simulink model "test_direct"  (R2024a)
settings: Solver=VariableStepAuto  StartTime=0.0  StopTime=40  RelTol=1e-3
libraries: neural x733, simulink x4
(part 8 of 35)

== system test_direct/Function Fitting Neural Network/Layer 4/Delays 1 ==
  "p{4}" : Inport  PortDimensions=20
      mask Display: e = 0.06;c1 = [120 230 180]/255;c2 = ([120 230 180]+0)/(256+128);c3 = ([120 230 180]+128)/(256+128);patch([0 1 1 0],[0 0 1 1],c1);patch([0 1 1 1-e 1-e 0+e],[0 0 1 1-e 0+e 0+e],c2);patch([0 0 1 1-e 0+e 0+e],[0 1 1 1-e 1-e 0+e],c3);plot([0 1 1 0 0],[0 0 1 1 0]);
  mux : Mux  Inputs=1
      mask Display: e = 0.06;c1 = [120 150 230]/255;c2 = ([120 150 230]+0)/383;c3 = ([120 150 230]+128)/383;patch([0 1 1 0],[0 0 1 1],c1);patch([0 1 1 1-e 1-e 0+e],[0 0 1 1-e 0+e 0+e],c2);patch([0 0 1 1-e 0+e 0+e],[0 1 1 1-e 1-e 0+e],c3);plot([0 1 1 0 0],[0 0 1 1 0]);disp('Mux')
  "pd{4,3}" : Outport
      mask Display: e = 0.06;c1 = [120 230 180]/255;c2 = ([120 230 180]+0)/(256+128);c3 = ([120 230 180]+128)/(256+128);patch([0 1 1 0],[0 0 1 1],c1);patch([0 1 1 1-e 1-e 0+e],[0 0 1 1-e 0+e 0+e],c2);patch([0 0 1 1-e 0+e 0+e],[0 1 1 1-e 1-e 0+e],c3);plot([0 1 1 0 0],[0 0 1 1 0]);
  wires:
  "p{4}"/1 -> mux/1
  mux/1 -> "pd{4,3}"/1

== system test_direct/Function Fitting Neural Network/Layer 4/LW{4,3} ==
  "ad{4,3}" : Inport  PortDimensions=20
      mask Display: e = 0.06;c1 = [120 230 180]/255;c2 = ([120 230 180]+0)/(256+128);c3 = ([120 230 180]+128)/(256+128);patch([0 1 1 0],[0 0 1 1],c1);patch([0 1 1 1-e 1-e 0+e],[0 0 1 1-e 0+e 0+e],c2);patch([0 0 1 1-e 0+e 0+e],[0 1 1 1-e 1-e 0+e],c3);plot([0 1 1 0 0],[0 0 1 1 0]);
  "IW{4,3}(1,:)'" : Constant  Value=[-0.0182808475685428926948983274769489071331918239593505859375;0.0804580234912133374081122383358888328075408935546875;-0.2073100011052473601314005691165220923721790313720703125;-0.56877624107405078124344299794756807386875152587890625;-0.37106551095573958587436891320976428687572479248046875;0.2453467469113256027579694773521623574197292327880859375;-0.1097157740776300016705135931260883808135986328125;0.293030747380307599048165911881369538605213165283203125;0.4286556952932023545344009107793681323528289794921875;-0.2927619933728118351012881248607300221920013427734375;-0.330831802187190826547436017790460027754306793212890625;-0.01300416253790542993329371057598109473474323749542236328125;-0.220024597925029985479028482586727477610111236572265625;0.28856741284184350693209353266865946352481842041015625;0.1738140495019694087286410422166227363049983978271484375;0.57653717402246307255353485743398778140544891357421875;-0.08144393527626341000580367790462332777678966522216796875;0.62386015914583803354531710283481515944004058837890625;0.23299635893419512466806509110028855502605438232421875;0.462827846568813539018805158775649033486843109130859375]
      mask Display: e = 0.06;c1 = [120 150 230]/255;c2 = ([120 150 230]+0)/383;c3 = ([120 150 230]+128)/383;patch([0 1 1 0],[0 0 1 1],c1);patch([0 1 1 1-e 1-e 0+e],[0 0 1 1-e 0+e 0+e],c2);patch([0 0 1 1-e 0+e 0+e],[0 1 1 1-e 1-e 0+e],c3);plot([0 1 1 0 0],[0 0 1 1 0]);disp('weights');
  "IW{4,3}(10,:)'" : Constant  Value=[-0.5867021051616487792301768422476015985012054443359375;-0.40646884911088843050919194865855388343334197998046875;0.1384930279966194444085658687981776893138885498046875;0.60431005202610743598512499374919570982456207275390625;0.231549088394502333709823460594634525477886199951171875;-0.278578383513912342106522146423230879008769989013671875;-0.2401723445859841599148154500653618015348911285400390625;-0.278682695857914330961335735992179252207279205322265625;0.389949189397055973049788235584856010973453521728515625;-0.378849241372464284882681795352254994213581085205078125;-0.50446895043893802412782179089845158159732818603515625;-0.04123499520558514264134686300167231820523738861083984375;-0.412512646032147267671774670816375873982906341552734375;0.0298074784018579376498880861845464096404612064361572265625;-0.6030020171920196236925448829424567520618438720703125;-0.0918971849790183037409718735943897627294063568115234375;-0.1048877360115925416739202091775950975716114044189453125;0.426138672134914464617594376250053755939006805419921875;-0.028373006982034938705528048785708961077034473419189453125;-0.10103546567123274091404283581141498871147632598876953125]
      mask Display: e = 0.06;c1 = [120 150 230]/255;c2 = ([120 150 230]+0)/383;c3 = ([120 150 230]+128)/383;patch([0 1 1 0],[0 0 1 1],c1);patch([0 1 1 1-e 1-e 0+e],[0 0 1 1-e 0+e 0+e],c2);patch([0 0 1 1-e 0+e 0+e],[0 1 1 1-e 1-e 0+e],c3);plot([0 1 1 0 0],[0 0 1 1 0]);disp('weights');
  "IW{4,3}(2,:)'" : Constant  Value=[0.04766233737430193573292314113132306374609470367431640625;0.472662950403235637697463289441657252609729766845703125;0.393481975518174265094017982846708036959171295166015625;-0.4054200644776970730021048439084552228450775146484375;0.64596436275341506672020841506309807300567626953125;0.34833116550052078963517487864010035991668701171875;0.0158927016381227755037475191102203098125755786895751953125;0.1432191124397620696218069724636734463274478912353515625;-0.1525863659129366445288411568981246091425418853759765625;-0.08213514792309771495038006605682312510907649993896484375;-0.05352653335257491484799885483880643732845783233642578125;-0.2237879229032577743652154822484590113162994384765625;-0.251639048104404128292088671514648012816905975341796875;0.374060271638200159127762844946119002997875213623046875;-0.13843849114586415094407811920973472297191619873046875;-0.00157935386633405584581868463800446988898329436779022216796875;0.08123459901137251859548626953255734406411647796630859375;-0.60194027599860344679427726077847182750701904296875;-0.2419573839009540316968838169486843980848789215087890625;0.4202479369474840797948900217306800186634063720703125]
      mask Display: e = 0.06;c1 = [120 150 230]/255;c2 = ([120 150 230]+0)/383;c3 = ([120 150 230]+128)/383;patch([0 1 1 0],[0 0 1 1],c1);patch([0 1 1 1-e 1-e 0+e],[0 0 1 1-e 0+e 0+e],c2);patch([0 0 1 1-e 0+e 0+e],[0 1 1 1-e 1-e 0+e],c3);plot([0 1 1 0 0],[0 0 1 1 0]);disp('weights');
  "IW{4,3}(3,:)'" : Constant  Value=[0.64653136532270083502993429647176526486873626708984375;-0.17598643231509558670921933298814110457897186279296875;-0.3306166204372065209327047341503202915191650390625;0.5500686330664434908754856223822571337223052978515625;-0.258915156366846421764904562223819084465503692626953125;-0.2135157354375183669237259209694457240402698516845703125;0.0280209258454371910873614837100831209681928157806396484375;0.023128965179387513118047792204379220493137836456298828125;0.300633725443321286885378640363342128694057464599609375;0.34519443371440450274434397215372882783412933349609375;-0.307061664525679400838953370111994445323944091796875;0.0201426192713053155147751027698177495039999485015869140625;0.1928095450190112358779259693619678728282451629638671875;-0.2828180192111175994540417377720586955547332763671875;0.67880942307011460368215693961246870458126068115234375;-0.18199528762274497228901282142032869160175323486328125;0.15160314165136490327512319709057919681072235107421875;0.48788420536031595897696888641803525388240814208984375;0.1995805530883998091251640971677261404693126678466796875;-0.39812724429761658928583756278385408222675323486328125]
      mask Display: e = 0.06;c1 = [120 150 230]/255;c2 = ([120 150 230]+0)/383;c3 = ([120 150 230]+128)/383;patch([0 1 1 0],[0 0 1 1],c1);patch([0 1 1 1-e 1-e 0+e],[0 0 1 1-e 0+e 0+e],c2);patch([0 0 1 1-e 0+e 0+e],[0 1 1 1-e 1-e 0+e],c3);plot([0 1 1 0 0],[0 0 1 1 0]);disp('weights');
  "IW{4,3}(4,:)'" : Constant  Value=[0.46897639649297795383375841993256472051143646240234375;0.1353316784521863269663555229271878488361835479736328125;-0.4090318643737698156570559149258770048618316650390625;-0.10034667176648993935916820419151918031275272369384765625;0.15356197843960306403943150144186802208423614501953125;-0.74982192036332262485842647947720251977443695068359375;0.736163475218127860699723896686919033527374267578125;-0.388099606476475178507001828620559535920619964599609375;0.1284378189965413030737551025595166720449924468994140625;-0.35342224141770184342448146708193235099315643310546875;0.33768468281888275317470515801687724888324737548828125;-0.33768459631601943637946305898367427289485931396484375;0.339246448835974323543496211641468107700347900390625;-0.182148817954333519519849460266414098441600799560546875;-0.45675022943742826786461819210671819746494293212890625;-0.1308331396638943433519131076536723412573337554931640625;0.007235920518857773438281544287065116805024445056915283203125;-0.2181989741993194120706078820148832164704799652099609375;0.697710740419517083665823520277626812458038330078125;0.03270757109621826030920743733076960779726505279541015625]
      mask Display: e = 0.06;c1 = [120 150 230]/255;c2 = ([120 150 230]+0)/383;c3 = ([120 150 230]+128)/383;patch([0 1 1 0],[0 0 1 1],c1);patch([0 1 1 1-e 1-e 0+e],[0 0 1 1-e 0+e 0+e],c2);patch([0 0 1 1-e 0+e 0+e],[0 1 1 1-e 1-e 0+e],c3);plot([0 1 1 0 0],[0 0 1 1 0]);disp('weights');
  "IW{4,3}(5,:)'" : Constant  Value=[0.254012415241254452258345963855390436947345733642578125;-0.278201611801674075774570837893406860530376434326171875;-0.130987915740999272262712338488199748098850250244140625;0.65659498971948615508864577350323088467121124267578125;-0.37010577209780526342086659496999345719814300537109375;-0.364239904557088711722911966717219911515712738037109375;-0.346218175332081823381003005124512128531932830810546875;-0.131514115645591733727570726841804571449756622314453125;-0.16293218459890457250338613448548130691051483154296875;-0.07690950801719813323398255988649907521903514862060546875;-0.04995568746558680384151074349574628286063671112060546875;-0.297894174787131815751450858442694880068302154541015625;-0.208190351516119920294300982277491129934787750244140625;-0.13629072817438714348980965951341204345226287841796875;-0.384110184134717147497184441817807964980602264404296875;-0.43900730118536801516171408366062678396701812744140625;0.0692901289663383213035530161505448631942272186279296875;0.27697027123827278050072209225618280470371246337890625;0.0208057391676239288036409647020263946615159511566162109375;0.6856311827603163155941956574679352343082427978515625]
      mask Display: e = 0.06;c1 = [120 150 230]/255;c2 = ([120 150 230]+0)/383;c3 = ([120 150 230]+128)/383;patch([0 1 1 0],[0 0 1 1],c1);patch([0 1 1 1-e 1-e 0+e],[0 0 1 1-e 0+e 0+e],c2);patch([0 0 1 1-e 0+e 0+e],[0 1 1 1-e 1-e 0+e],c3);plot([0 1 1 0 0],[0 0 1 1 0]);disp('weights');
  "IW{4,3}(6,:)'" : Constant  Value=[0.06383515321962386634968567022951901890337467193603515625;-0.348969499010585881837442912001279182732105255126953125;-0.67269644646642923202506381130660884082317352294921875;0.44685601061213520157622269834973849356174468994140625;-0.358281232233862712011074336260207928717136383056640625;0.07916658582745154937310161358254845254123210906982421875;0.30505773608176711686468252082704566419124603271484375;0.617951579143801499327537385397590696811676025390625;-0.25294218554518221875326844383380375802516937255859375;-0.3977997598759459574324637287645600736141204833984375;0.058739564042513479902307693691909662447869777679443359375;0.1494537664697459522500366801978088915348052978515625;0.60851330942889114705707243047072552144527435302734375;-0.055559362022579848738867980273425928317010402679443359375;-0.62443423379172180442964190660859458148479461669921875;-0.2268644620133335454426060096011497080326080322265625;-0.57816378248105604331641416138154454529285430908203125;0.39207408987547409662255404327879659831523895263671875;-0.074342103653326108148036155398585833609104156494140625;0.285697237530900871593786405355785973370075225830078125]
      mask Display: e = 0.06;c1 = [120 150 230]/255;c2 = ([120 150 230]+0)/383;c3 = ([120 150 230]+128)/383;patch([0 1 1 0],[0 0 1 1],c1);patch([0 1 1 1-e 1-e 0+e],[0 0 1 1-e 0+e 0+e],c2);patch([0 0 1 1-e 0+e 0+e],[0 1 1 1-e 1-e 0+e],c3);plot([0 1 1 0 0],[0 0 1 1 0]);disp('weights');
  "IW{4,3}(7,:)'" : Constant  Value=[0.1735578250848583692356186247707228176295757293701171875;-0.1443796965013408317712872985794092528522014617919921875;-0.00192713703805364963174417969327123500988818705081939697265625;-0.050944766962450170610932076442622928880155086517333984375;-0.56313960947635821607804018640308640897274017333984375;0.406795735506861155794666728979791514575481414794921875;-0.43477191912486556901740186731331050395965576171875;-0.0183635163924778209432187026095562032423913478851318359375;-0.16499808196158738393677367639611475169658660888671875;0.1554097258561016603461979457279085181653499603271484375;-0.45712271023931894120551078231073915958404541015625;-0.31639810290967407269135946989990770816802978515625;0.283675985048455980841453083485248498618602752685546875;-0.434852696669257132722208325503743253648281097412109375;0.184268928265691245282908994340687058866024017333984375;0.487799544058790834899497212973074056208133697509765625;-0.1646897501250245976489594568192842416465282440185546875;0.55969685707381255923564822296611964702606201171875;-0.40425367209081686237226449520676396787166595458984375;0.259423740372571154377823177128448151051998138427734375]
      mask Display: e = 0.06;c1 = [120 150 230]/255;c2 = ([120 150 230]+0)/383;c3 = ([120 150 230]+128)/383;patch([0 1 1 0],[0 0 1 1],c1);patch([0 1 1 1-e 1-e 0+e],[0 0 1 1-e 0+e 0+e],c2);patch([0 0 1 1-e 0+e 0+e],[0 1 1 1-e 1-e 0+e],c3);plot([0 1 1 0 0],[0 0 1 1 0]);disp('weights');
  "IW{4,3}(8,:)'" : Constant  Value=[-0.044604630833756091223829542968815076164901256561279296875;0.1653273492054885551727494430451770313084125518798828125;0.35228947713259184393308487415197305381298065185546875;0.388185803066177392839364301835303194820880889892578125;0.59881679713870406001063884104951284825801849365234375;-0.07736001152979880834958947843915666453540325164794921875;-0.5271011175306501428394767572171986103057861328125;-0.09774032952107626626148118020864785648882389068603515625;0.18675638954029449845251065198681317269802093505859375;-0.478571423377917526398306335977395065128803253173828125;0.34027059434836159912407538286061026155948638916015625;0.057705036219698628563445907957429881207644939422607421875;-0.214782881199087782864154405615408904850482940673828125;-0.26706306507587018739258155619609169661998748779296875;-0.54002602442711433727851044750423170626163482666015625;0.58528571806826767964793134524370543658733367919921875;0.030194751746646243673044551769635290838778018951416015625;-0.4346282259921803170499288171413354575634002685546875;0.40357189348227062719587365791085176169872283935546875;0.193904249336287748395335484019597060978412628173828125]
      mask Display: e = 0.06;c1 = [120 150 230]/255;c2 = ([120 150 230]+0)/383;c3 = ([120 150 230]+128)/383;patch([0 1 1 0],[0 0 1 1],c1);patch([0 1 1 1-e 1-e 0+e],[0 0 1 1-e 0+e 0+e],c2);patch([0 0 1 1-e 0+e 0+e],[0 1 1 1-e 1-e 0+e],c3);plot([0 1 1 0 0],[0 0 1 1 0]);disp('weights');
  "IW{4,3}(9,:)'" : Constant  Value=[-0.262696724536377546055376797085045836865901947021484375;-0.495272708083491608466175648572971113026142120361328125;-0.3543852059837149237608855401049368083477020263671875;-0.221393523730061769771992885580402798950672149658203125;-0.038436478394411034698041618185015977360308170318603515625;-0.318611608590077199920642669894732534885406494140625;-0.07339652443837078876764934420862118713557720184326171875;1.061095964250348355761843777145259082317352294921875;-0.4127361165109009188967092995881102979183197021484375;-0.025399426654827285398940972527270787395536899566650390625;-0.5236953508005728341601070496835745871067047119140625;-0.335822568857687187016125562877277843654155731201171875;0.350185935701288586496815469217835925519466400146484375;-0.195141267318745648129407754822750575840473175048828125;0.9131446131154741241431338494294323027133941650390625;-0.4326775227891754838083215872757136821746826171875;-0.63697775880777218748818313542869873344898223876953125;0.55100216042612715217074992324342019855976104736328125;-0.09919080628567943092033232233006856404244899749755859375;0.134968530413840992476792735033086501061916351318359375]
      mask Display: e = 0.06;c1 = [120 150 230]/255;c2 = ([120 150 230]+0)/383;c3 = ([120 150 230]+128)/383;patch([0 1 1 0],[0 0 1 1],c1);patch([0 1 1 1-e 1-e 0+e],[0 0 1 1-e 0+e 0+e],c2);patch([0 0 1 1-e 0+e 0+e],[0 1 1 1-e 1-e 0+e],c3);plot([0 1 1 0 0],[0 0 1 1 0]);disp('weights');
  Mux : Mux  Inputs=10
      mask Display: e = 0.06;c1 = [120 150 230]/255;c2 = ([120 150 230]+0)/383;c3 = ([120 150 230]+128)/383;patch([0 1 1 0],[0 0 1 1],c1);patch([0 1 1 1-e 1-e 0+e],[0 0 1 1-e 0+e 0+e],c2);patch([0 0 1 1-e 0+e 0+e],[0 1 1 1-e 1-e 0+e],c3);plot([0 1 1 0 0],[0 0 1 1 0]);disp('Mux');
  dotprod{1..10} (10 alike) : neural/Weight Functions/dotprod
  "lz{4,3}" : Outport
      mask Display: e = 0.06;c1 = [120 230 180]/255;c2 = ([120 230 180]+0)/(256+128);c3 = ([120 230 180]+128)/(256+128);patch([0 1 1 0],[0 0 1 1],c1);patch([0 1 1 1-e 1-e 0+e],[0 0 1 1-e 0+e 0+e],c2);patch([0 0 1 1-e 0+e 0+e],[0 1 1 1-e 1-e 0+e],c3);plot([0 1 1 0 0],[0 0 1 1 0]);
  wires:
  "IW{4,3}(1,:)'"/1 -> dotprod1/1
  "ad{4,3}"/1 -> dotprod1/2, dotprod2/2, dotprod3/2, dotprod4/2, dotprod5/2, dotprod6/2, dotprod7/2, dotprod8/2, dotprod9/2, dotprod10/2
  dotprod1/1 -> Mux/1
  "IW{4,3}(2,:)'"/1 -> dotprod2/1
  dotprod2/1 -> Mux/2
  "IW{4,3}(3,:)'"/1 -> dotprod3/1
  dotprod3/1 -> Mux/3
  "IW{4,3}(4,:)'"/1 -> dotprod4/1
  dotprod4/1 -> Mux/4
  "IW{4,3}(5,:)'"/1 -> dotprod5/1
  dotprod5/1 -> Mux/5
  "IW{4,3}(6,:)'"/1 -> dotprod6/1
  dotprod6/1 -> Mux/6
  "IW{4,3}(7,:)'"/1 -> dotprod7/1
  dotprod7/1 -> Mux/7
  "IW{4,3}(8,:)'"/1 -> dotprod8/1
  dotprod8/1 -> Mux/8
  "IW{4,3}(9,:)'"/1 -> dotprod9/1
  dotprod9/1 -> Mux/9
  "IW{4,3}(10,:)'"/1 -> dotprod10/1
  dotprod10/1 -> Mux/10
  Mux/1 -> "lz{4,3}"/1

== system test_direct/Function Fitting Neural Network/Layer 5/Delays 1 ==
  "p{5}" : Inport  PortDimensions=10
      mask Display: e = 0.06;c1 = [120 230 180]/255;c2 = ([120 230 180]+0)/(256+128);c3 = ([120 230 180]+128)/(256+128);patch([0 1 1 0],[0 0 1 1],c1);patch([0 1 1 1-e 1-e 0+e],[0 0 1 1-e 0+e 0+e],c2);patch([0 0 1 1-e 0+e 0+e],[0 1 1 1-e 1-e 0+e],c3);plot([0 1 1 0 0],[0 0 1 1 0]);
  mux : Mux  Inputs=1
      mask Display: e = 0.06;c1 = [120 150 230]/255;c2 = ([120 150 230]+0)/383;c3 = ([120 150 230]+128)/383;patch([0 1 1 0],[0 0 1 1],c1);patch([0 1 1 1-e 1-e 0+e],[0 0 1 1-e 0+e 0+e],c2);patch([0 0 1 1-e 0+e 0+e],[0 1 1 1-e 1-e 0+e],c3);plot([0 1 1 0 0],[0 0 1 1 0]);disp('Mux')
  "pd{5,4}" : Outport
      mask Display: e = 0.06;c1 = [120 230 180]/255;c2 = ([120 230 180]+0)/(256+128);c3 = ([120 230 180]+128)/(256+128);patch([0 1 1 0],[0 0 1 1],c1);patch([0 1 1 1-e 1-e 0+e],[0 0 1 1-e 0+e 0+e],c2);patch([0 0 1 1-e 0+e 0+e],[0 1 1 1-e 1-e 0+e],c3);plot([0 1 1 0 0],[0 0 1 1 0]);
  wires:
  "p{5}"/1 -> mux/1
  mux/1 -> "pd{5,4}"/1

== system test_direct/Function Fitting Neural Network/Layer 5/LW{5,4} ==
  "ad{5,4}" : Inport  PortDimensions=10
      mask Display: e = 0.06;c1 = [120 230 180]/255;c2 = ([120 230 180]+0)/(256+128);c3 = ([120 230 180]+128)/(256+128);patch([0 1 1 0],[0 0 1 1],c1);patch([0 1 1 1-e 1-e 0+e],[0 0 1 1-e 0+e 0+e],c2);patch([0 0 1 1-e 0+e 0+e],[0 1 1 1-e 1-e 0+e],c3);plot([0 1 1 0 0],[0 0 1 1 0]);
  "IW{5,4}(1,:)'" : Constant  Value=[-0.609586613853234648985335297766141593456268310546875;-0.991992343621268535258650445030070841312408447265625;0.55645920623334166332796257847803644835948944091796875;-0.2756548382209949021870443175430409610271453857421875;0.79182679604217509616859160814783535897731781005859375;0.5409353217326822171884259660146199166774749755859375;0.8560146531317720519638214682345278561115264892578125;0.369094621261524424848943226606934331357479095458984375;1.144450010398711636838697813800536096096038818359375;0.82688754328264491011424297539633698761463165283203125]
      mask Display: e = 0.06;c1 = [120 150 230]/255;c2 = ([120 150 230]+0)/383;c3 = ([120 150 230]+128)/383;patch([0 1 1 0],[0 0 1 1],c1);patch([0 1 1 1-e 1-e 0+e],[0 0 1 1-e 0+e 0+e],c2);patch([0 0 1 1-e 0+e 0+e],[0 1 1 1-e 1-e 0+e],c3);plot([0 1 1 0 0],[0 0 1 1 0]);disp('weights');
  "IW{5,4}(2,:)'" : Constant  Value=[-0.2491134788551136736156621509508113376796245574951171875;-0.348638402621329834829566607368178665637969970703125;-0.58928454736647262190984974949969910085201263427734375;1.1057017527083596863946013399981893599033355712890625;0.69839147102565746205726782136480323970317840576171875;-0.78717405206411239504404875333420932292938232421875;0.1763952297557981607756261155373067595064640045166015625;-0.0641150518456101436992611297682742588222026824951171875;-0.9062580556750947646804661417263559997081756591796875;-1.0565207862803387417471867593121714890003204345703125]
      mask Display: e = 0.06;c1 = [120 150 230]/255;c2 = ([120 150 230]+0)/383;c3 = ([120 150 230]+128)/383;patch([0 1 1 0],[0 0 1 1],c1);patch([0 1 1 1-e 1-e 0+e],[0 0 1 1-e 0+e 0+e],c2);patch([0 0 1 1-e 0+e 0+e],[0 1 1 1-e 1-e 0+e],c3);plot([0 1 1 0 0],[0 0 1 1 0]);disp('weights');
  Mux : Mux  Inputs=2
      mask Display: e = 0.06;c1 = [120 150 230]/255;c2 = ([120 150 230]+0)/383;c3 = ([120 150 230]+128)/383;patch([0 1 1 0],[0 0 1 1],c1);patch([0 1 1 1-e 1-e 0+e],[0 0 1 1-e 0+e 0+e],c2);patch([0 0 1 1-e 0+e 0+e],[0 1 1 1-e 1-e 0+e],c3);plot([0 1 1 0 0],[0 0 1 1 0]);disp('Mux');
  dotprod1 : neural/Weight Functions/dotprod
  dotprod2 : neural/Weight Functions/dotprod
  "lz{5,4}" : Outport
      mask Display: e = 0.06;c1 = [120 230 180]/255;c2 = ([120 230 180]+0)/(256+128);c3 = ([120 230 180]+128)/(256+128);patch([0 1 1 0],[0 0 1 1],c1);patch([0 1 1 1-e 1-e 0+e],[0 0 1 1-e 0+e 0+e],c2);patch([0 0 1 1-e 0+e 0+e],[0 1 1 1-e 1-e 0+e],c3);plot([0 1 1 0 0],[0 0 1 1 0]);
  wires:
  "IW{5,4}(1,:)'"/1 -> dotprod1/1
  "ad{5,4}"/1 -> dotprod1/2, dotprod2/2
  dotprod1/1 -> Mux/1
  "IW{5,4}(2,:)'"/1 -> dotprod2/1
  dotprod2/1 -> Mux/2
  Mux/1 -> "lz{5,4}"/1

== system test_direct/Function Fitting Neural Network1/Layer 1/Delays 1 ==
  "p{1}" : Inport  PortDimensions=8
      mask Display: e = 0.06;c1 = [120 230 180]/255;c2 = ([120 230 180]+0)/(256+128);c3 = ([120 230 180]+128)/(256+128);patch([0 1 1 0],[0 0 1 1],c1);patch([0 1 1 1-e 1-e 0+e],[0 0 1 1-e 0+e 0+e],c2);patch([0 0 1 1-e 0+e 0+e],[0 1 1 1-e 1-e 0+e],c3);plot([0 1 1 0 0],[0 0 1 1 0]);
  mux : Mux  Inputs=1
      mask Display: e = 0.06;c1 = [120 150 230]/255;c2 = ([120 150 230]+0)/383;c3 = ([120 150 230]+128)/383;patch([0 1 1 0],[0 0 1 1],c1);patch([0 1 1 1-e 1-e 0+e],[0 0 1 1-e 0+e 0+e],c2);patch([0 0 1 1-e 0+e 0+e],[0 1 1 1-e 1-e 0+e],c3);plot([0 1 1 0 0],[0 0 1 1 0]);disp('Mux')
  "pd{1,1}" : Outport
      mask Display: e = 0.06;c1 = [120 230 180]/255;c2 = ([120 230 180]+0)/(256+128);c3 = ([120 230 180]+128)/(256+128);patch([0 1 1 0],[0 0 1 1],c1);patch([0 1 1 1-e 1-e 0+e],[0 0 1 1-e 0+e 0+e],c2);patch([0 0 1 1-e 0+e 0+e],[0 1 1 1-e 1-e 0+e],c3);plot([0 1 1 0 0],[0 0 1 1 0]);
  wires:
  "p{1}"/1 -> mux/1
  mux/1 -> "pd{1,1}"/1

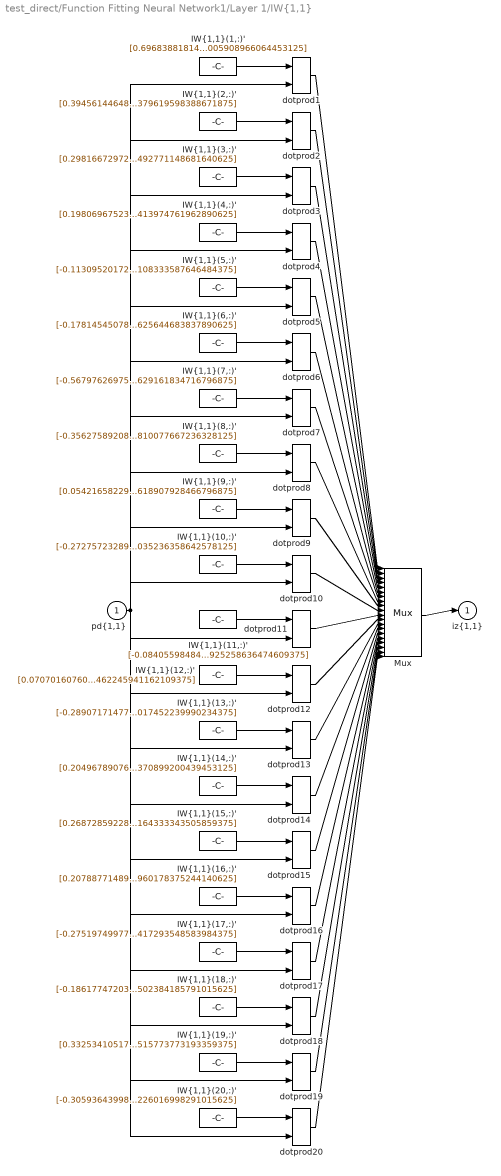
== system test_direct/Function Fitting Neural Network1/Layer 1/IW{1,1} ==
  "pd{1,1}" : Inport  PortDimensions=8
      mask Display: e = 0.06;c1 = [120 230 180]/255;c2 = ([120 230 180]+0)/(256+128);c3 = ([120 230 180]+128)/(256+128);patch([0 1 1 0],[0 0 1 1],c1);patch([0 1 1 1-e 1-e 0+e],[0 0 1 1-e 0+e 0+e],c2);patch([0 0 1 1-e 0+e 0+e],[0 1 1 1-e 1-e 0+e],c3);plot([0 1 1 0 0],[0 0 1 1 0]);
  "IW{1,1}(1,:)'" : Constant  Value=[0.69683881814263559650868273820378817617893218994140625;0.7640431505441267479028510933858342468738555908203125;0.67792814742460449917160758559475652873516082763671875;-0.564455292301047517611323200981132686138153076171875;0.0206524861164411911718108427749029942788183689117431640625;0.63667859510223190344646582161658443510532379150390625;1.00234633248641813452195492573082447052001953125;0.05889755968272869512958322957274504005908966064453125]
      mask Display: e = 0.06;c1 = [120 150 230]/255;c2 = ([120 150 230]+0)/383;c3 = ([120 150 230]+128)/383;patch([0 1 1 0],[0 0 1 1],c1);patch([0 1 1 1-e 1-e 0+e],[0 0 1 1-e 0+e 0+e],c2);patch([0 0 1 1-e 0+e 0+e],[0 1 1 1-e 1-e 0+e],c3);plot([0 1 1 0 0],[0 0 1 1 0]);disp('Weights');
  "IW{1,1}(10,:)'" : Constant  Value=[-0.272757232895687706797360760901938192546367645263671875;-0.26724039829289625291863785605528391897678375244140625;0.07275557598798353120539417204781784676015377044677734375;-0.2024513959855038514046299269466544501483440399169921875;0.3419638465162890827997443921049125492572784423828125;1.33460318464404448235427480540238320827484130859375;-0.0387887916615675398812612684196210466325283050537109375;0.213400994483100625576099673708085902035236358642578125]
      mask Display: e = 0.06;c1 = [120 150 230]/255;c2 = ([120 150 230]+0)/383;c3 = ([120 150 230]+128)/383;patch([0 1 1 0],[0 0 1 1],c1);patch([0 1 1 1-e 1-e 0+e],[0 0 1 1-e 0+e 0+e],c2);patch([0 0 1 1-e 0+e 0+e],[0 1 1 1-e 1-e 0+e],c3);plot([0 1 1 0 0],[0 0 1 1 0]);disp('Weights');
  "IW{1,1}(11,:)'" : Constant  Value=[-0.08405598484492704525194994857884012162685394287109375;0.22475151025755268907602157923975028097629547119140625;0.515237557803050805205202777869999408721923828125;0.362218047367421858151459446162334643304347991943359375;0.6853072384581058162922317933407612144947052001953125;0.49951312939876679752870813899789936840534210205078125;0.30454149529149532327210181392729282379150390625;-1.2259255997811100424854657831019721925258636474609375]
      mask Display: e = 0.06;c1 = [120 150 230]/255;c2 = ([120 150 230]+0)/383;c3 = ([120 150 230]+128)/383;patch([0 1 1 0],[0 0 1 1],c1);patch([0 1 1 1-e 1-e 0+e],[0 0 1 1-e 0+e 0+e],c2);patch([0 0 1 1-e 0+e 0+e],[0 1 1 1-e 1-e 0+e],c3);plot([0 1 1 0 0],[0 0 1 1 0]);disp('Weights');
  "IW{1,1}(12,:)'" : Constant  Value=[0.070701607607360938967389074605307541787624359130859375;0.360937305657575258077685020907665602862834930419921875;-0.54966145677578925887729610622045584022998809814453125;0.57478890048600173034998306320630945265293121337890625;0.5999359439613123345935719044064171612262725830078125;-0.1187698884370364804663466884449007920920848846435546875;-0.98272714657886572897638188806013204157352447509765625;0.3155743205749350632771665914333425462245941162109375]
      mask Display: e = 0.06;c1 = [120 150 230]/255;c2 = ([120 150 230]+0)/383;c3 = ([120 150 230]+128)/383;patch([0 1 1 0],[0 0 1 1],c1);patch([0 1 1 1-e 1-e 0+e],[0 0 1 1-e 0+e 0+e],c2);patch([0 0 1 1-e 0+e 0+e],[0 1 1 1-e 1-e 0+e],c3);plot([0 1 1 0 0],[0 0 1 1 0]);disp('Weights');
  "IW{1,1}(13,:)'" : Constant  Value=[-0.2890717147788859353596535584074445068836212158203125;-0.242197251466092222660364541297894902527332305908203125;0.1863621649756492526517348551351460628211498260498046875;0.5305730473676708580654803881770931184291839599609375;-0.410514280193981451194673581994720734655857086181640625;-0.32544911037928070385305545642040669918060302734375;-0.1853150999010389210486238198427599854767322540283203125;1.117782813867628899373585227294825017452239990234375]
      mask Display: e = 0.06;c1 = [120 150 230]/255;c2 = ([120 150 230]+0)/383;c3 = ([120 150 230]+128)/383;patch([0 1 1 0],[0 0 1 1],c1);patch([0 1 1 1-e 1-e 0+e],[0 0 1 1-e 0+e 0+e],c2);patch([0 0 1 1-e 0+e 0+e],[0 1 1 1-e 1-e 0+e],c3);plot([0 1 1 0 0],[0 0 1 1 0]);disp('Weights');
  "IW{1,1}(14,:)'" : Constant  Value=[0.20496789076231902715363730749231763184070587158203125;0.26429751124447797838712403972749598324298858642578125;0.36484988902725346004984885439625941216945648193359375;-0.5745167996217379613455022990819998085498809814453125;-0.497719456328582554593964459854760207235813140869140625;1.2500259012874488373512349426164291799068450927734375;0.159100403766398112992419555666856467723846435546875;-1.011690432173470544086057998356409370899200439453125]
      mask Display: e = 0.06;c1 = [120 150 230]/255;c2 = ([120 150 230]+0)/383;c3 = ([120 150 230]+128)/383;patch([0 1 1 0],[0 0 1 1],c1);patch([0 1 1 1-e 1-e 0+e],[0 0 1 1-e 0+e 0+e],c2);patch([0 0 1 1-e 0+e 0+e],[0 1 1 1-e 1-e 0+e],c3);plot([0 1 1 0 0],[0 0 1 1 0]);disp('Weights');
  "IW{1,1}(15,:)'" : Constant  Value=[0.268728592282806710844766939771943725645542144775390625;0.3038613381826598125456939669675193727016448974609375;0.289458329765824140533680974840535782277584075927734375;-0.5409659514970897031815866284887306392192840576171875;-0.341031491431749878007195775353466160595417022705078125;0.289089703738018399814535541736404411494731903076171875;-1.0600111717134639288673270129947923123836517333984375;-0.283062967641139306973485645357868634164333343505859375]
      mask Display: e = 0.06;c1 = [120 150 230]/255;c2 = ([120 150 230]+0)/383;c3 = ([120 150 230]+128)/383;patch([0 1 1 0],[0 0 1 1],c1);patch([0 1 1 1-e 1-e 0+e],[0 0 1 1-e 0+e 0+e],c2);patch([0 0 1 1-e 0+e 0+e],[0 1 1 1-e 1-e 0+e],c3);plot([0 1 1 0 0],[0 0 1 1 0]);disp('Weights');
  "IW{1,1}(16,:)'" : Constant  Value=[0.2078877148940026231560551650545676238834857940673828125;0.0840721456582262105516889505452127195894718170166015625;0.4795104000373415775726471110829152166843414306640625;-0.767481223732529027614646111032925546169281005859375;0.45378680057911624512456683078198693692684173583984375;-1.107609818954824465464525928837247192859649658203125;0.0561311271008308187990820670165703631937503814697265625;1.3254891299923559078166590552427805960178375244140625]
      mask Display: e = 0.06;c1 = [120 150 230]/255;c2 = ([120 150 230]+0)/383;c3 = ([120 150 230]+128)/383;patch([0 1 1 0],[0 0 1 1],c1);patch([0 1 1 1-e 1-e 0+e],[0 0 1 1-e 0+e 0+e],c2);patch([0 0 1 1-e 0+e 0+e],[0 1 1 1-e 1-e 0+e],c3);plot([0 1 1 0 0],[0 0 1 1 0]);disp('Weights');
  "IW{1,1}(17,:)'" : Constant  Value=[-0.275197499773989162630272176102153025567531585693359375;-0.44914330240078592648700350764556787908077239990234375;-0.10215451095910664525145961079033440910279750823974609375;-0.336551936442363419654810741121764294803142547607421875;0.1538071143495922943333908960994449444115161895751953125;-0.86003499709754260837968331543379463255405426025390625;-1.1816622408107642083763266782625578343868255615234375;0.6442531105253210821359743931679986417293548583984375]
      mask Display: e = 0.06;c1 = [120 150 230]/255;c2 = ([120 150 230]+0)/383;c3 = ([120 150 230]+128)/383;patch([0 1 1 0],[0 0 1 1],c1);patch([0 1 1 1-e 1-e 0+e],[0 0 1 1-e 0+e 0+e],c2);patch([0 0 1 1-e 0+e 0+e],[0 1 1 1-e 1-e 0+e],c3);plot([0 1 1 0 0],[0 0 1 1 0]);disp('Weights');
  "IW{1,1}(18,:)'" : Constant  Value=[-0.18617747203861301219518509242334403097629547119140625;0.6961684748736256533874211527290754020214080810546875;-0.794298894762984541983996678027324378490447998046875;0.9533966695713740335804686765186488628387451171875;-0.429132320048394466649455125661916099488735198974609375;-0.60641702663512209170448841177858412265777587890625;-0.5869788837731719777224270728765986859798431396484375;-0.67739230044078679870978021426708437502384185791015625]
      mask Display: e = 0.06;c1 = [120 150 230]/255;c2 = ([120 150 230]+0)/383;c3 = ([120 150 230]+128)/383;patch([0 1 1 0],[0 0 1 1],c1);patch([0 1 1 1-e 1-e 0+e],[0 0 1 1-e 0+e 0+e],c2);patch([0 0 1 1-e 0+e 0+e],[0 1 1 1-e 1-e 0+e],c3);plot([0 1 1 0 0],[0 0 1 1 0]);disp('Weights');
  "IW{1,1}(19,:)'" : Constant  Value=[0.332534105179708106003744205736438743770122528076171875;0.1373651819662270179289720317683531902730464935302734375;-0.095512741275323442824429776010219939053058624267578125;-0.92288801670492404127799090929329395294189453125;0.6482460639796414625379838980734348297119140625;0.359576586366763761848375224872143007814884185791015625;0.06857172282922495420987019087988301180303096771240234375;1.3221821932444155489605464026681147515773773193359375]
      mask Display: e = 0.06;c1 = [120 150 230]/255;c2 = ([120 150 230]+0)/383;c3 = ([120 150 230]+128)/383;patch([0 1 1 0],[0 0 1 1],c1);patch([0 1 1 1-e 1-e 0+e],[0 0 1 1-e 0+e 0+e],c2);patch([0 0 1 1-e 0+e 0+e],[0 1 1 1-e 1-e 0+e],c3);plot([0 1 1 0 0],[0 0 1 1 0]);disp('Weights');
  "IW{1,1}(2,:)'" : Constant  Value=[0.394561446481398292451814313608338125050067901611328125;0.496126296863468263520502432584180496633052825927734375;0.456100600010595214062192326309741474688053131103515625;-0.628533744301563501721830107271671295166015625;-0.7743125299354953749997321210685186088085174560546875;1.2798934719664074588507673979620449244976043701171875;0.78492340665270976529654944897629320621490478515625;-0.433530743610808400045897315067122690379619598388671875]
      mask Display: e = 0.06;c1 = [120 150 230]/255;c2 = ([120 150 230]+0)/383;c3 = ([120 150 230]+128)/383;patch([0 1 1 0],[0 0 1 1],c1);patch([0 1 1 1-e 1-e 0+e],[0 0 1 1-e 0+e 0+e],c2);patch([0 0 1 1-e 0+e 0+e],[0 1 1 1-e 1-e 0+e],c3);plot([0 1 1 0 0],[0 0 1 1 0]);disp('Weights');
  "IW{1,1}(20,:)'" : Constant  Value=[-0.30593643998864517019597997204982675611972808837890625;-0.9213158914543253530382571625523269176483154296875;0.7853169865737832378016491929884068667888641357421875;-0.81818362218703821753251759218983352184295654296875;-0.56443628264250544912528084751102142035961151123046875;-0.56868329177563092802216715426766313612461090087890625;-0.32446229273851467933553749389830045402050018310546875;-0.94825291764287611417927337242872454226016998291015625]
      mask Display: e = 0.06;c1 = [120 150 230]/255;c2 = ([120 150 230]+0)/383;c3 = ([120 150 230]+128)/383;patch([0 1 1 0],[0 0 1 1],c1);patch([0 1 1 1-e 1-e 0+e],[0 0 1 1-e 0+e 0+e],c2);patch([0 0 1 1-e 0+e 0+e],[0 1 1 1-e 1-e 0+e],c3);plot([0 1 1 0 0],[0 0 1 1 0]);disp('Weights');
  "IW{1,1}(3,:)'" : Constant  Value=[0.298166729727484425271910595256485976278781890869140625;-0.4183300027243743723914803922525607049465179443359375;-0.80799038393734090579556550437700934708118438720703125;-0.505366820627469959248401210061274468898773193359375;-0.253730462639679188452390690144966356456279754638671875;0.83661243378666227954454370774328708648681640625;-0.78793602729768352777028894706745631992816925048828125;-0.8556624788960223160216855831095017492771148681640625]
      mask Display: e = 0.06;c1 = [120 150 230]/255;c2 = ([120 150 230]+0)/383;c3 = ([120 150 230]+128)/383;patch([0 1 1 0],[0 0 1 1],c1);patch([0 1 1 1-e 1-e 0+e],[0 0 1 1-e 0+e 0+e],c2);patch([0 0 1 1-e 0+e 0+e],[0 1 1 1-e 1-e 0+e],c3);plot([0 1 1 0 0],[0 0 1 1 0]);disp('Weights');
  "IW{1,1}(4,:)'" : Constant  Value=[0.1980696752360057433239859392415382899343967437744140625;0.2404467731306450251071993307050433941185474395751953125;0.1788655051560224806816989939761697314679622650146484375;-0.3289918451008759792131286303629167377948760986328125;0.1697279131019995279672230026335455477237701416015625;-0.437020546507040308359393065984477289021015167236328125;1.00415962486495136118946902570314705371856689453125;1.0487130245760918345609979951404966413974761962890625]
      mask Display: e = 0.06;c1 = [120 150 230]/255;c2 = ([120 150 230]+0)/383;c3 = ([120 150 230]+128)/383;patch([0 1 1 0],[0 0 1 1],c1);patch([0 1 1 1-e 1-e 0+e],[0 0 1 1-e 0+e 0+e],c2);patch([0 0 1 1-e 0+e 0+e],[0 1 1 1-e 1-e 0+e],c3);plot([0 1 1 0 0],[0 0 1 1 0]);disp('Weights');
  "IW{1,1}(5,:)'" : Constant  Value=[-0.1130952017268885001488598618379910476505756378173828125;0.1344070985514231042490251866183825768530368804931640625;-0.76878839995911640858849978030775673687458038330078125;0.297090955023965985759559771395288407802581787109375;0.52419815521998902596578773227520287036895751953125;-0.405912798675867769748748514757608063519001007080078125;0.9627247316031388724155704039731062948703765869140625;0.1682518404063882699883691884679137729108333587646484375]
      mask Display: e = 0.06;c1 = [120 150 230]/255;c2 = ([120 150 230]+0)/383;c3 = ([120 150 230]+128)/383;patch([0 1 1 0],[0 0 1 1],c1);patch([0 1 1 1-e 1-e 0+e],[0 0 1 1-e 0+e 0+e],c2);patch([0 0 1 1-e 0+e 0+e],[0 1 1 1-e 1-e 0+e],c3);plot([0 1 1 0 0],[0 0 1 1 0]);disp('Weights');
  "IW{1,1}(6,:)'" : Constant  Value=[-0.1781454507860589508982940287751262076199054718017578125;0.004443753562727384594233104309068949078209698200225830078125;-0.69841504074740334839788147291983477771282196044921875;0.7818190218670781899135135972755961120128631591796875;-0.04258378226915589259693462054201518185436725616455078125;0.5771509638363261363025458194897510111331939697265625;1.012078828578088174339200122631154954433441162109375;0.38439957448017347818591815666877664625644683837890625]
      mask Display: e = 0.06;c1 = [120 150 230]/255;c2 = ([120 150 230]+0)/383;c3 = ([120 150 230]+128)/383;patch([0 1 1 0],[0 0 1 1],c1);patch([0 1 1 1-e 1-e 0+e],[0 0 1 1-e 0+e 0+e],c2);patch([0 0 1 1-e 0+e 0+e],[0 1 1 1-e 1-e 0+e],c3);plot([0 1 1 0 0],[0 0 1 1 0]);disp('Weights');
  "IW{1,1}(7,:)'" : Constant  Value=[-0.567976269758097895845594393904320895671844482421875;-0.62358958862428937042210463914670981466770172119140625;1.1372939244395856572822367525077424943447113037109375;0.79605135173232943746057799216941930353641510009765625;-0.283657482715290287789144940688856877386569976806640625;-0.159043735376311001772364761563949286937713623046875;-0.0593283380696205397963893801716039888560771942138671875;0.381766617901312332872265642436104826629161834716796875]
      mask Display: e = 0.06;c1 = [120 150 230]/255;c2 = ([120 150 230]+0)/383;c3 = ([120 150 230]+128)/383;patch([0 1 1 0],[0 0 1 1],c1);patch([0 1 1 1-e 1-e 0+e],[0 0 1 1-e 0+e 0+e],c2);patch([0 0 1 1-e 0+e 0+e],[0 1 1 1-e 1-e 0+e],c3);plot([0 1 1 0 0],[0 0 1 1 0]);disp('Weights');
  "IW{1,1}(8,:)'" : Constant  Value=[-0.356275892087113188466673818766139447689056396484375;-0.439399300119033553446712403456331230700016021728515625;0.469170009999208215134558486170135438442230224609375;0.3747641605057603353401418644352816045284271240234375;0.25274429229424300036299655403126962482929229736328125;-0.11199155851085661195210008145295432768762111663818359375;0.057299253967103717932740636342714424245059490203857421875;1.10880888617612516355848129023797810077667236328125]
      mask Display: e = 0.06;c1 = [120 150 230]/255;c2 = ([120 150 230]+0)/383;c3 = ([120 150 230]+128)/383;patch([0 1 1 0],[0 0 1 1],c1);patch([0 1 1 1-e 1-e 0+e],[0 0 1 1-e 0+e 0+e],c2);patch([0 0 1 1-e 0+e 0+e],[0 1 1 1-e 1-e 0+e],c3);plot([0 1 1 0 0],[0 0 1 1 0]);disp('Weights');
  "IW{1,1}(9,:)'" : Constant  Value=[0.05421658229498470260576681312159053049981594085693359375;-0.03453621247591280585265138824979658238589763641357421875;0.064985110646265720202308102670940570533275604248046875;-0.260421675482414405333742024595267139375209808349609375;-0.01956377235233054678875674881055601872503757476806640625;-0.242897431994648471675901646449347026646137237548828125;-0.76987318408289506788122480429592542350292205810546875;1.11916213564057187568323570303618907928466796875]
      mask Display: e = 0.06;c1 = [120 150 230]/255;c2 = ([120 150 230]+0)/383;c3 = ([120 150 230]+128)/383;patch([0 1 1 0],[0 0 1 1],c1);patch([0 1 1 1-e 1-e 0+e],[0 0 1 1-e 0+e 0+e],c2);patch([0 0 1 1-e 0+e 0+e],[0 1 1 1-e 1-e 0+e],c3);plot([0 1 1 0 0],[0 0 1 1 0]);disp('Weights');
  Mux : Mux  Inputs=20
      mask Display: e = 0.06;c1 = [120 150 230]/255;c2 = ([120 150 230]+0)/383;c3 = ([120 150 230]+128)/383;patch([0 1 1 0],[0 0 1 1],c1);patch([0 1 1 1-e 1-e 0+e],[0 0 1 1-e 0+e 0+e],c2);patch([0 0 1 1-e 0+e 0+e],[0 1 1 1-e 1-e 0+e],c3);plot([0 1 1 0 0],[0 0 1 1 0]);disp('Mux');
  dotprod{1..20} (20 alike) : neural/Weight Functions/dotprod
  "iz{1,1}" : Outport
      mask Display: e = 0.06;c1 = [120 230 180]/255;c2 = ([120 230 180]+0)/(256+128);c3 = ([120 230 180]+128)/(256+128);patch([0 1 1 0],[0 0 1 1],c1);patch([0 1 1 1-e 1-e 0+e],[0 0 1 1-e 0+e 0+e],c2);patch([0 0 1 1-e 0+e 0+e],[0 1 1 1-e 1-e 0+e],c3);plot([0 1 1 0 0],[0 0 1 1 0]);
  wires:
  "IW{1,1}(1,:)'"/1 -> dotprod1/1
  "pd{1,1}"/1 -> dotprod1/2, dotprod2/2, dotprod3/2, dotprod4/2, dotprod5/2, dotprod6/2, dotprod7/2, dotprod8/2, dotprod9/2, dotprod10/2, dotprod11/2, dotprod12/2, dotprod13/2, dotprod14/2, dotprod15/2, dotprod16/2, dotprod17/2, dotprod18/2, dotprod19/2, dotprod20/2
  dotprod1/1 -> Mux/1
  "IW{1,1}(2,:)'"/1 -> dotprod2/1
  dotprod2/1 -> Mux/2
  "IW{1,1}(3,:)'"/1 -> dotprod3/1
  dotprod3/1 -> Mux/3
  "IW{1,1}(4,:)'"/1 -> dotprod4/1
  dotprod4/1 -> Mux/4
  "IW{1,1}(5,:)'"/1 -> dotprod5/1
  dotprod5/1 -> Mux/5
  "IW{1,1}(6,:)'"/1 -> dotprod6/1
  dotprod6/1 -> Mux/6
  "IW{1,1}(7,:)'"/1 -> dotprod7/1
  dotprod7/1 -> Mux/7
  "IW{1,1}(8,:)'"/1 -> dotprod8/1
  dotprod8/1 -> Mux/8
  "IW{1,1}(9,:)'"/1 -> dotprod9/1
  dotprod9/1 -> Mux/9
  "IW{1,1}(10,:)'"/1 -> dotprod10/1
  dotprod10/1 -> Mux/10
  "IW{1,1}(11,:)'"/1 -> dotprod11/1
  dotprod11/1 -> Mux/11
  "IW{1,1}(12,:)'"/1 -> dotprod12/1
  dotprod12/1 -> Mux/12
  "IW{1,1}(13,:)'"/1 -> dotprod13/1
  dotprod13/1 -> Mux/13
  "IW{1,1}(14,:)'"/1 -> dotprod14/1
  dotprod14/1 -> Mux/14
  "IW{1,1}(15,:)'"/1 -> dotprod15/1
  dotprod15/1 -> Mux/15
  "IW{1,1}(16,:)'"/1 -> dotprod16/1
  dotprod16/1 -> Mux/16
  "IW{1,1}(17,:)'"/1 -> dotprod17/1
  dotprod17/1 -> Mux/17
  "IW{1,1}(18,:)'"/1 -> dotprod18/1
  dotprod18/1 -> Mux/18
  "IW{1,1}(19,:)'"/1 -> dotprod19/1
  dotprod19/1 -> Mux/19
  "IW{1,1}(20,:)'"/1 -> dotprod20/1
  dotprod20/1 -> Mux/20
  Mux/1 -> "iz{1,1}"/1

== system test_direct/Function Fitting Neural Network1/Layer 2/Delays 1 ==
  "p{2}" : Inport  PortDimensions=20
      mask Display: e = 0.06;c1 = [120 230 180]/255;c2 = ([120 230 180]+0)/(256+128);c3 = ([120 230 180]+128)/(256+128);patch([0 1 1 0],[0 0 1 1],c1);patch([0 1 1 1-e 1-e 0+e],[0 0 1 1-e 0+e 0+e],c2);patch([0 0 1 1-e 0+e 0+e],[0 1 1 1-e 1-e 0+e],c3);plot([0 1 1 0 0],[0 0 1 1 0]);
  mux : Mux  Inputs=1
      mask Display: e = 0.06;c1 = [120 150 230]/255;c2 = ([120 150 230]+0)/383;c3 = ([120 150 230]+128)/383;patch([0 1 1 0],[0 0 1 1],c1);patch([0 1 1 1-e 1-e 0+e],[0 0 1 1-e 0+e 0+e],c2);patch([0 0 1 1-e 0+e 0+e],[0 1 1 1-e 1-e 0+e],c3);plot([0 1 1 0 0],[0 0 1 1 0]);disp('Mux')
  "pd{2,1}" : Outport
      mask Display: e = 0.06;c1 = [120 230 180]/255;c2 = ([120 230 180]+0)/(256+128);c3 = ([120 230 180]+128)/(256+128);patch([0 1 1 0],[0 0 1 1],c1);patch([0 1 1 1-e 1-e 0+e],[0 0 1 1-e 0+e 0+e],c2);patch([0 0 1 1-e 0+e 0+e],[0 1 1 1-e 1-e 0+e],c3);plot([0 1 1 0 0],[0 0 1 1 0]);
  wires:
  "p{2}"/1 -> mux/1
  mux/1 -> "pd{2,1}"/1
